simulink model "power_seriesload"  (Simulink 6.0)
settings: Solver=ode23s  SolverMode=SingleTasking  StartTime=0.0  StopTime=0.1  RelTol=1e-3  AbsTol=1e-6
libraries: powerlib x8
settings Model: Creator=patrice  LastModifiedBy=batserve  ExtModeTrigMode=oneshot  ExtModeArmWhenConnect=off  ExtModeAutoUpdateStatusClock=off
settings DataIOCC: LimitDataPoints=off  SignalLoggingName=sigsOut
settings OptimizationCC: BooleanDataType=off
settings DebuggingCC: SolverPrmCheckMsg=none
settings HardwareCC: TargetUnknown=on
settings RTWCC: TemplateMakefile=grt_unix.tmf

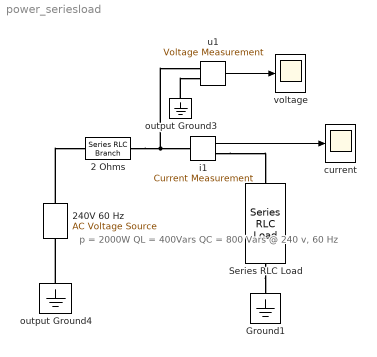
== system power_seriesload ==
  note: p = 2000W
      | QL = 400Vars
      | QC = 800 Vars
      | @ 240 v, 60 Hz
  2 Ohms : powerlib/Elements/Series RLC Branch  PhysicalDomain=powersysdomain  SubClassName=unknown  PortType=p1  LConnTagsString=__new0  RConnTagsString=__new0  Resistance=2  Inductance=0  Capacitance=inf  Measurements=None
  240V 60 Hz : powerlib/Electrical Sources/AC Voltage Source  Description=source block  Orientation=up  Amplitude=240  Phase=0  Frequency=60  SampleTime=0  Measurements=None
      settings: AttributesFormatString=\n
  Ground1 : powerlib/Elements/Ground  Orientation=down  PhysicalDomain=powersysdomain  SubClassName=unknown  PortType=p1  LConnTagsString=a
  "Series RLC Load " : powerlib/Elements/Series RLC Load  Orientation=down  PhysicalDomain=powersysdomain  SubClassName=unknown  PortType=p1  LConnTagsString=a  RConnTagsString=__new0  NominalVoltage=240  NominalFrequency=60  ActivePower=2000  InductivePower=400  CapacitivePower=800  Measurements=None
  current : Scope
      settings: TickLabels=on  TimeRange=0.1  YMin=-15  YMax=15  DataFormat=Array
  i1 : powerlib/Measurements/Current Measurement  Tag=PoWeRsYsTeMmEaSuReMeNt  PhasorSimulation=off  OutputType=Magnitude  PSBequivalent=0
  output Ground3 : powerlib/Elements/Ground  Orientation=down  PhysicalDomain=powersysdomain  SubClassName=unknown  PortType=p1  LConnTagsString=a
  output Ground4 : powerlib/Elements/Ground  Orientation=down  PhysicalDomain=powersysdomain  SubClassName=unknown  PortType=p1  LConnTagsString=a
  u1 : powerlib/Measurements/Voltage Measurement  Tag=PoWeRsYsTeMmEaSuReMeNt  PhasorSimulation=off  OutputType=Magnitude  PSBequivalent=0
  voltage : Scope
      settings: TickLabels=on  TimeRange=0.1  YMin=-400  YMax=400  DataFormat=Array
  wires:
  u1/1 -> voltage/1
  i1/1 -> current/1
  connections:
  240V 60 Hz/RConn1 -- 2 Ohms/LConn1
  output Ground4/LConn1 -- 240V 60 Hz/LConn1
  output Ground3/LConn1 -- u1/LConn2
  2 Ohms/RConn1 -- u1/LConn1 -- i1/LConn1
  i1/RConn1 -- "Series RLC Load "/LConn1
  "Series RLC Load "/RConn1 -- Ground1/LConn1
